simulink model "MPC"  (R2018a)
settings: Solver=VariableStepAuto  StartTime=0.0  StopTime=18  FixedStep=0.01  RelTol=1e-3
PreLoadFcn:
  | setUpPurePursuitCurveHighVel
model workspace (MAT data in the model file):
  firstWarning = 0
  originalScenarioChecksum = 'F73A6DA3C723D3CA73A6F931B7A52A9C'
values from neighbouring files (symbols this model uses):
  mu = m    [PSO_MPC.m]
  ref = i    [PSO_MPC.m]
  vx = j    [PSO_MPC.m]
  wy = l    [PSO_MPC.m]
undefined symbols (not defined in the file or in its folder): parms
libraries: autolibutils x4, autolibshared x3, vehdynlibviscommon x1, simulink x1
(part 1 of 3)
settings Model: PacingRate=0.700000  Creator=valakshe  LastModifiedBy=yassi
settings DataIOCC: ReturnWorkspaceOutputs=on
settings SFSimCC: SimUseLocalCustomCode=on
settings RTWCC: RTWUseLocalCustomCode=on

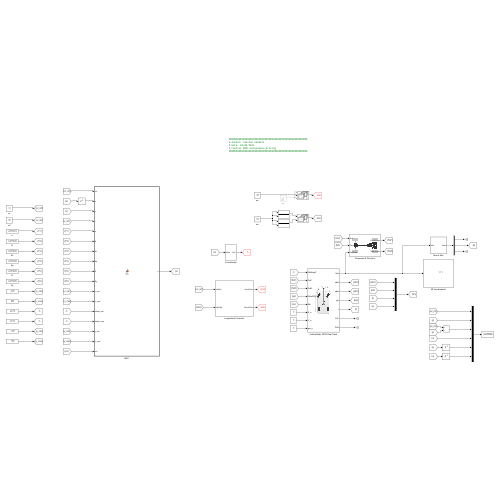
[thumbnail: Simulink's stored preview of the top-level diagram]
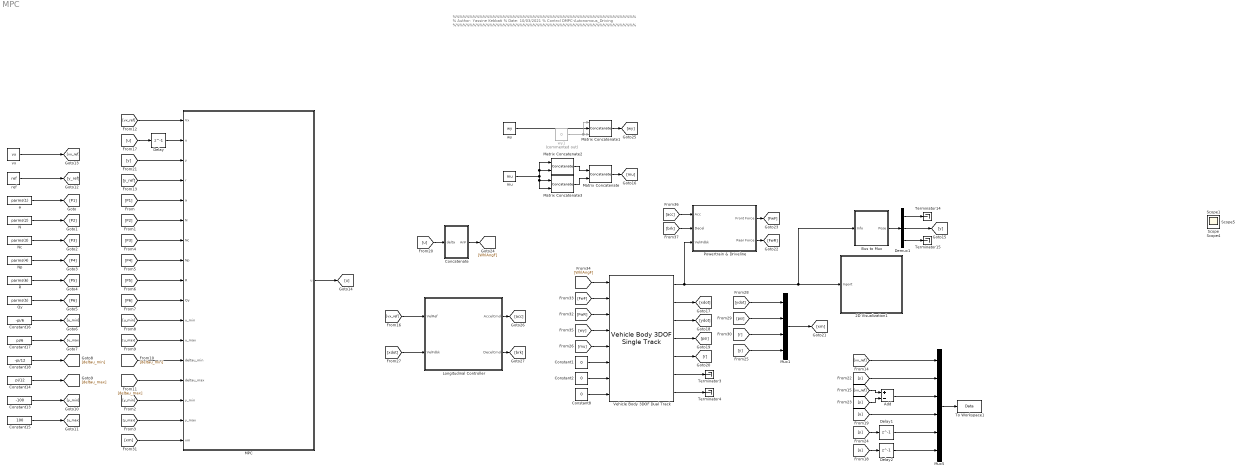
== system MPC ==
  note: %%%%%%%%%%%%%%%%%%%%%%%%%%%%%%%%%%%%%%%%%%%%%%%%%%%%%%%
      | % Author: Yassine Kebbati
      | % Date: 10/03/2021
      | % Control DMPC-Autonomous_Driving
      | %%%%%%%%%%%%%%%%%%%%%%%%%%%%%%%%%%%%%%%%%%%%%%%%%%%%%%%
  2D Visualization1 : Subsystem
      mask Display: image("visualization.JPG");
  Add : Sum  Inputs=+-
  Bus to Mux : Subsystem
  Concatenate : Subsystem
  Constant1 : Constant  Value=0
  Constant13 : Constant  Value=-100
  Constant14 : Constant  Value=pi/12
  Constant15 : Constant  Value=100
  Constant16 : Constant  Value=-pi/6
  Constant17 : Constant  Value=pi/6
  Constant18 : Constant  Value=-pi/12
  Constant2 : Constant  Value=0
  Constant8 : Constant  Value=0
  Delay : Delay  DelayLength=1
  Delay1 : Delay  DelayLength=1
  Delay2 : Delay  DelayLength=1
  Demux1 : Demux  Outputs=3
  Longitudinal Controller : Subsystem
  MPC : MATLAB Function  TreatAsAtomicUnit=on
  Matrix Concatenate : Concatenate  Mode=Multidimensional array  ConcatenateDimension=2
  Matrix Concatenate1 : Concatenate  NumInputs=3  Mode=Multidimensional array  ConcatenateDimension=2
  Matrix Concatenate2 : Concatenate  ConcatenateDimension=2
  Matrix Concatenate3 : Concatenate  ConcatenateDimension=2
  Mux1 : Mux
  Mux5 : Mux  Inputs=6
  N : Constant  Value=parms(2)
  Nc : Constant  Value=parms(3)
  Np : Constant  Value=parms(4)
  Powertrain & Driveline : Subsystem
      mask Display: image('vdbslibpt.png');
  Qy : Constant  Value=parms(5)
  R : Constant  Value=parms(6)
  Terminator{3..4,14..15} (4 alike) : Terminator
  To Workspace1 : ToWorkspace  VariableName=Data  SaveFormat=Timeseries  SampleTime=-1
  Vehicle Body 3DOF Dual Track : autolibshared/Vehicle Body 3DOF Single Track  trackMode=Dual  inputMode=External longitudinal forces  frontSteerMode=on  rearSteerMode=off  windMode=on  muMode=on  extFMode=off  extMMode=off  htchFMode=off  htchMMode=off  aMode=2  NF=2  NR=2  m=1575  a=1.2  b=1.6  h=0.35  dh=1  hh=0.2  X_o=0  xdot_o=0  CalphaMode=off  sigmaMode=on  hl=0  w=[1.4,1.4]  Cy_f=19e3  Cy_r=33e3  sigma_f=.1  sigma_r=.1  alpha_f_brk=[-.1 .1]  Cy_f_data=[-9e3 9e3]  alpha_r_brk=[-.1 .1]  Cy_r_data=[-9e3 9e3]  Y_o=0  ydot_o=0  Izz=2875  psi_o=0  r_o=0  Af=2  Cd=.3  Cl=.1  Cpm=.1  beta_w=[0:0.01:0.3]  Cs=[0:0.03:0.9]  Cym=[0:0.01:0.3]  Pabs=101325  Tair=273  g=9.81  mu=1  xdot_tol=0.01  Fznom=5000  Fxtire_sat=7e4  Fytire_sat=7e4
  a : Constant  Value=parms(1)
  mu : Constant  Value=mu
  ref : Constant  Value=ref
  vx : Constant  Value=vx
  wy : Constant  Value=wy
  wy1 : Constant  Commented=on  Value=0
  Scope{,1,4..5} (4 alike) : Scope
  wires:
  Vehicle Body 3DOF Dual Track/7 -> Terminator4/1
  Constant1/1 -> Vehicle Body 3DOF Dual Track/6
  Vehicle Body 3DOF Dual Track/6 -> Terminator3/1
  Constant2/1 -> Vehicle Body 3DOF Dual Track/7
  Constant8/1 -> Vehicle Body 3DOF Dual Track/8
  Vehicle Body 3DOF Dual Track/1 -> 2D Visualization1/1(Inport), Bus to Mux/1(Info), Powertrain & Driveline/3(VehFdbk)
  [acc] -> Powertrain & Driveline/1(Acc)
  [brk] -> Powertrain & Driveline/2(Decel)
  Vehicle Body 3DOF Dual Track/2 -> [xdot]
  Vehicle Body 3DOF Dual Track/4 -> [psi]
  Vehicle Body 3DOF Dual Track/5 -> [r]
  [P5] -> MPC/9(R)
  [P1] -> MPC/5(a)
  [P4] -> MPC/8(Np)
  [u_min] -> MPC/11(u_min)
  [deltau_min] -> MPC/13(deltau_min)
  [P3] -> MPC/7(Nc)
  [y_min] -> MPC/15(y_min)
  [y_max] -> MPC/16(y_max)
  Delay/1 -> MPC/2("u ")
  [deltau_max] -> MPC/14(deltau_max)
  [P2] -> MPC/6(N)
  [P6] -> MPC/10(Qy)
  [u_max] -> MPC/12(u_max)
  Demux1/3 -> Terminator15/1
  Demux1/1 -> Terminator14/1
  Vehicle Body 3DOF Dual Track/3 -> [ydot]
  Add/1 -> Mux5/3
  Mux5/1 -> To Workspace1/1
  Bus to Mux/1(Pose) -> Demux1/1
  Concatenate/1(AnF) -> [WhlAngF]
  wy/1 -> Matrix Concatenate1/2
  wy1/1 -> Matrix Concatenate1/1, Matrix Concatenate1/3
  Matrix Concatenate2/1 -> Matrix Concatenate/1
  mu/1 -> Matrix Concatenate2/1, Matrix Concatenate2/2, Matrix Concatenate3/1, Matrix Concatenate3/2
  Matrix Concatenate3/1 -> Matrix Concatenate/2
  Delay1/1 -> Mux5/5
  Delay2/1 -> Mux5/6
  Demux1/2 -> [y]
  a/1 -> [P1]
  N/1 -> [P2]
  Nc/1 -> [P3]
  Np/1 -> [P4]
  R/1 -> [P5]
  Qy/1 -> [P6]
  Constant16/1 -> [u_min]
  Constant17/1 -> [u_max]
  Constant18/1 -> [deltau_min]
  Constant14/1 -> [deltau_max]
  Constant13/1 -> [y_min]
  Constant15/1 -> [y_max]
  ref/1 -> [y_ref]
  vx/1 -> [vx_ref]
  [vx_ref] -> MPC/1(Vx)
  [y_ref] -> MPC/4(r)
  [vx_ref] -> Mux5/1
  [vx_ref] -> Add/1
  [vx_ref] -> Longitudinal Controller/1(VelRef)
  MPC/1(u) -> [u]
  [u] -> Delay/1
  [u] -> Delay2/1
  [u] -> Mux5/4
  [u] -> Concatenate/1(delta)
  [y] -> MPC/3(y)
  [y] -> Mux5/2
  [y] -> Add/2
  [y] -> Delay1/1
  [xdot] -> Longitudinal Controller/2(VelFdbk)
  [xm] -> MPC/17(xm)
  [psi] -> Mux1/2
  Mux1/1 -> [xm]
  [ydot] -> Mux1/1
  [r] -> Mux1/3
  [y] -> Mux1/4
  Powertrain & Driveline/2(Rear Force) -> [FwR]
  Powertrain & Driveline/1(Front Force) -> [FwF]
  [FwF] -> Vehicle Body 3DOF Dual Track/2
  [FwR] -> Vehicle Body 3DOF Dual Track/3
  [WhlAngF] -> Vehicle Body 3DOF Dual Track/1
  [mu] -> Vehicle Body 3DOF Dual Track/5
  Matrix Concatenate/1 -> [mu]
  [wy] -> Vehicle Body 3DOF Dual Track/4
  Matrix Concatenate1/1 -> [wy]
  Longitudinal Controller/1(AccelCmd) -> [acc]
  Longitudinal Controller/2(DecelCmd) -> [brk]

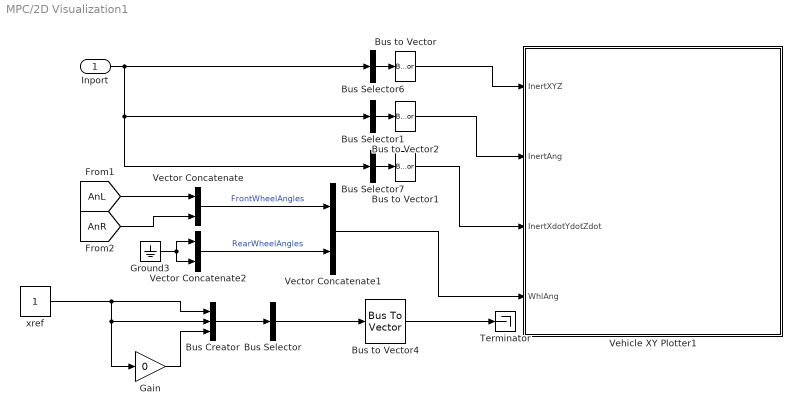
== system MPC/2D Visualization1 ==
  Inport : Inport
  Bus Creator : BusCreator  Inputs=3
  Bus Selector : BusSelector  OutputSignals=signal1,signal2,signal3  OutputAsBus=on
  Bus Selector1 : BusSelector  OutputSignals=InertFrm.Cg.Ang.phi,InertFrm.Cg.Ang.theta,InertFrm.Cg.Ang.psi  OutputAsBus=on
  Bus Selector6 : BusSelector  OutputSignals=InertFrm.Geom.Disp.X,InertFrm.Geom.Disp.Y,InertFrm.Geom.Disp.Z  OutputAsBus=on
  Bus Selector7 : BusSelector  OutputSignals=InertFrm.Geom.Vel.Xdot,InertFrm.Geom.Vel.Ydot,InertFrm.Geom.Vel.Zdot  OutputAsBus=on
  Bus to Vector{,1..2,4} (4 alike) : BusToVector
  Gain : Gain  Gain=0
  Ground3 : Ground
  Terminator : Terminator
  Vector Concatenate : Concatenate
  Vector Concatenate1 : Concatenate
  Vector Concatenate2 : Concatenate
  Vehicle XY Plotter1 : Subsystem  mask(Vehicle XY Plotter){extRef=off, extStats=off, extTireF=off, a=2, b=2, w=2, figBorder=10, bufferSize=1024, velNorm=5, tireFNorm=1000, pltDT=0.1}
      mask prompts: extRef "Plot path reference, extRef"; extStats "Display speed, RPM and Gear"; extTireF "Display tire forces"; a "Distance to front axle from CG, a [m]:"; b "Distance to rear axle from CG, b [m]:"; w "Track width, w [m]:"; figBorder "Distance to figure borders, figBorder [m]:"; bufferSize "Path buffer sampe size, bufferSize []:"; velNorm "Velocity vector scaling, velNorm [m*s/m]:"; tireFNorm "Tire force vector scaling, tireFNorm [m/N]:"; pltDT "Plot update rate, pltDT [s]:"
      mask help:
      | This block will display a MATLAB figure which indicates the vehicle path, current position and heading velocity.
      | An optional path reference is also provided.
      mask init:
      | block = gcb;
      | if autoblkschecksimstopped(block)
      |     ParamNames = {'extRef';'extStats';'extTireF';'extTireF'};
      |     PortNames = {'RefXYZ';'Stats';'TireFx';'TireFy'};
      |     for idx=1:length(PortNames)
      |         InportOption  = {'built-in/Ground', [PortNames{idx}, ' Ground'];...
      |             'built-in/Inport',PortNames{idx}};
      |         if ~strcmp(get_param(block,ParamNames{idx}),'on')
      |             NewBlkHdl = autoblksreplaceblock(block, InportOption, 1);
      |             set_param(NewBlkHdl, 'ShowName', 'off');
      |         else
      |             autoblksreplaceblock(block, InportOption, 2);
      |         end
      |     end
      |     InportNames = {'InertXYZ';'InertAng';'InertXdotYdotZdot';'WhlAng';'RefXYZ';'Stats';'TireFx';'TireFy'};
      |     FoundNames = get_param(find_system(block, 'LookUnderMasks', 'all', 'SearchDepth', 1, 'FollowLinks', 'on', 'BlockType', 'Inport'), 'Name');
      |     [~,PortI] = intersect(InportNames, FoundNames);
      |     PortI = sort(PortI);
      |     for idx = 1:length(PortI)
      |         set_param([block, '/', InportNames{PortI(idx)}], 'Port', num2str(idx));
      |     end
      | end
      mask TypeOptions a: Vehicle XY Plotter/a
      mask TypeOptions b: Vehicle XY Plotter/b
      mask TypeOptions w: Vehicle XY Plotter/w
      mask TypeOptions figBorder: Vehicle XY Plotter/figBorder
      mask TypeOptions bufferSize: Vehicle XY Plotter/bufferSize
      mask TypeOptions velNorm: Vehicle XY Plotter/velNorm
      mask TypeOptions tireFNorm: Vehicle XY Plotter/tireFNorm
      mask DialogControl Container3 Prompt: Plot and Display Options
  xref : Constant
  wires:
  Vector Concatenate1/1 -> Vehicle XY Plotter1/4(WhlAng)
  Ground3/1 -> Vector Concatenate2/1, Vector Concatenate2/2
  Bus Selector6/1 -> Bus to Vector/1
  Vector Concatenate/1 -> Vector Concatenate1/1  "FrontWheelAngles"
  [AnL] -> Vector Concatenate/1
  Vector Concatenate2/1 -> Vector Concatenate1/2  "RearWheelAngles"
  Bus Selector7/1 -> Bus to Vector1/1
  Bus to Vector1/1 -> Vehicle XY Plotter1/3(InertXdotYdotZdot)
  Bus to Vector/1 -> Vehicle XY Plotter1/1(InertXYZ)
  Bus to Vector2/1 -> Vehicle XY Plotter1/2(InertAng)
  Bus Selector1/1 -> Bus to Vector2/1
  [AnR] -> Vector Concatenate/2
  Inport/1 -> Bus Selector7/1, Bus Selector1/1, Bus Selector6/1
  Bus to Vector4/1 -> Terminator/1
  Bus Selector/1 -> Bus to Vector4/1
  xref/1 -> Gain/1, Bus Creator/2, Bus Creator/1
  Gain/1 -> Bus Creator/3
  Bus Creator/1 -> Bus Selector/1

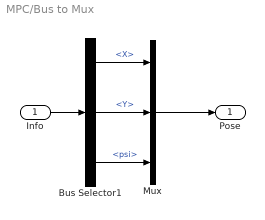
== system MPC/Bus to Mux ==
  Info : Inport
  Bus Selector1 : BusSelector  OutputSignals=InertFrm.Cg.Disp.X,InertFrm.Cg.Disp.Y,InertFrm.Cg.Ang.psi
  Mux : Mux  Inputs=3
  Pose : Outport
  wires:
  Bus Selector1/3 -> Mux/3  "<psi>"
  Bus Selector1/1 -> Mux/1  "<X>"
  Mux/1 -> Pose/1
  Bus Selector1/2 -> Mux/2  "<Y>"
  Info/1 -> Bus Selector1/1

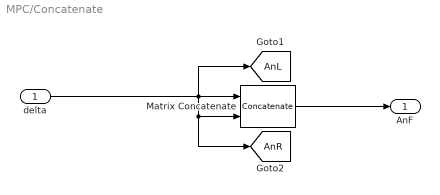
== system MPC/Concatenate ==
  delta : Inport
  Matrix Concatenate : Concatenate
  AnF : Outport  VectorParamsAs1DForOutWhenUnconnected=off
  tag scope: AnL=global, AnR=global
  wires:
  Matrix Concatenate/1 -> AnF/1
  delta/1 -> [AnL], [AnR], Matrix Concatenate/2, Matrix Concatenate/1

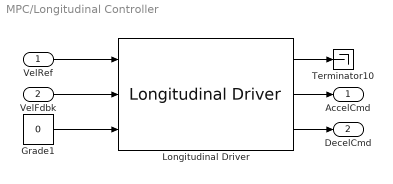
== system MPC/Longitudinal Controller ==
  VelRef : Inport
  VelFdbk : Inport  Port=2
  Grade1 : Constant  Value=0
  Longitudinal Driver : autolibshared/Longitudinal Driver  Kp=100  Ki=1  Kff=.1  Kg=0  vnom=9  Kaw=1  tauerr=.01  aMode=2
  Terminator10 : Terminator
  AccelCmd : Outport
  DecelCmd : Outport  Port=2
  wires:
  Grade1/1 -> Longitudinal Driver/3
  Longitudinal Driver/3 -> DecelCmd/1
  VelRef/1 -> Longitudinal Driver/1
  VelFdbk/1 -> Longitudinal Driver/2
  Longitudinal Driver/2 -> AccelCmd/1
  Longitudinal Driver/1 -> Terminator10/1

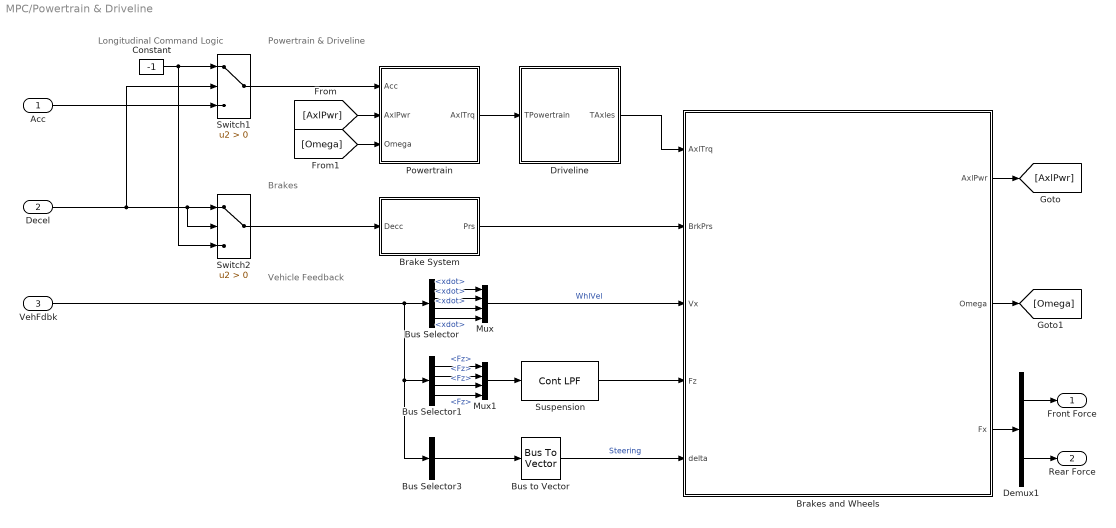
== system MPC/Powertrain & Driveline ==
  note: Vehicle Feedback
  note: Powertrain & Driveline
  note: Brakes
  note: Longitudinal Command Logic
  Acc : Inport
  Decel : Inport  Port=2
  VehFdbk : Inport  Port=3
  Brake System : Subsystem
  Brakes and Wheels : Subsystem  TreatAsAtomicUnit=on
      mask Display: image('vdbslibwhls.png');
  Bus Selector : BusSelector  OutputSignals=BdyFrm.FrntAxl.Lft.Vel.xdot,BdyFrm.FrntAxl.Rght.Vel.xdot,BdyFrm.RearAxl.Lft.Vel.xdot,BdyFrm.RearAxl.Rght.Vel.xdot
  Bus Selector1 : BusSelector  OutputSignals=BdyFrm.Forces.FrntAxl.Lft.Fz,BdyFrm.Forces.FrntAxl.Rght.Fz,BdyFrm.Forces.RearAxl.Lft.Fz,BdyFrm.Forces.RearAxl.Rght.Fz
  Bus Selector3 : BusSelector  OutputSignals=BdyFrm.FrntAxl.Steer.WhlAngFL,BdyFrm.FrntAxl.Steer.WhlAngFR,BdyFrm.RearAxl.Steer.WhlAngRL,BdyFrm.RearAxl.Steer.WhlAngRR  OutputAsBus=on
  Bus to Vector : BusToVector
  Constant : Constant  Value=-1
  Demux1 : Demux  Outputs=[2 2]
  Driveline : Subsystem  Variant=on  VariantControl=Variant1  OverrideUsingVariant=0
  Mux : Mux
  Mux1 : Mux
  Powertrain : Subsystem
  Suspension : autolibutils/Cont LPF  wc=10*pi*2  AbsoluteTolerance=auto  aMode=2
  Switch1 : Switch  Criteria=u2 > Threshold
  Switch2 : Switch  Criteria=u2 > Threshold
  Front Force : Outport  VectorParamsAs1DForOutWhenUnconnected=off
  Rear Force : Outport  Port=2  VectorParamsAs1DForOutWhenUnconnected=off
  wires:
  Brake System/1(Prs) -> Brakes and Wheels/2(BrkPrs)
  Switch2/1 -> Brake System/1(Decc)
  [Omega] -> Powertrain/3(Omega)
  [AxlPwr] -> Powertrain/2(AxlPwr)
  Brakes and Wheels/2(Omega) -> [Omega]
  Powertrain/1(AxlTrq) -> Driveline/1(TPowertrain)
  Switch1/1 -> Powertrain/1(Acc)
  Bus Selector1/4 -> Mux1/4  "<Fz>"
  Bus Selector1/3 -> Mux1/3  "<Fz>"
  Bus Selector1/2 -> Mux1/2  "<Fz>"
  Bus Selector1/1 -> Mux1/1  "<Fz>"
  Bus Selector/4 -> Mux/4  "<xdot>"
  Bus Selector/3 -> Mux/3  "<xdot>"
  Bus Selector/2 -> Mux/2  "<xdot>"
  Bus Selector/1 -> Mux/1  "<xdot>"
  Suspension/1 -> Brakes and Wheels/4(Fz)
  Mux1/1 -> Suspension/1
  Bus to Vector/1 -> Brakes and Wheels/5(delta)  "Steering"
  Bus Selector3/1 -> Bus to Vector/1
  Brakes and Wheels/3(Fx) -> Demux1/1
  Brakes and Wheels/1(AxlPwr) -> [AxlPwr]
  Driveline/1(TAxles) -> Brakes and Wheels/1(AxlTrq)
  Demux1/2 -> Rear Force/1
  Demux1/1 -> Front Force/1
  VehFdbk/1 -> Bus Selector/1, Bus Selector1/1, Bus Selector3/1
  Mux/1 -> Brakes and Wheels/3(Vx)  "WhlVel"
  Constant/1 -> Switch1/1, Switch2/3
  Acc/1 -> Switch1/3
  Decel/1 -> Switch2/1, Switch2/2, Switch1/2

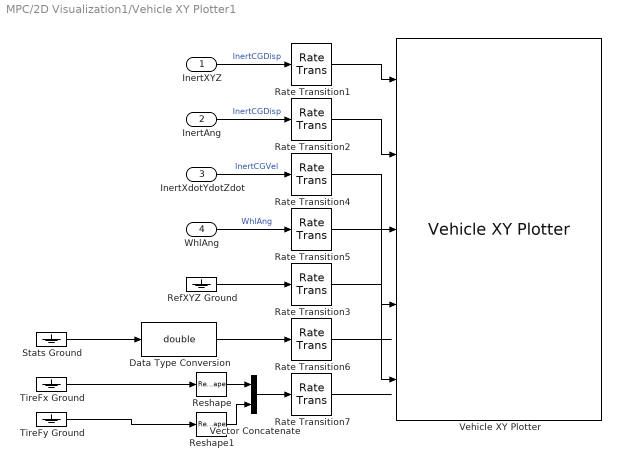
== system MPC/2D Visualization1/Vehicle XY Plotter1 ==
  InertXYZ : Inport
  InertAng : Inport  Port=2
  InertXdotYdotZdot : Inport  Port=3
  WhlAng : Inport  Port=4
  Data Type Conversion : DataTypeConversion  OutDataTypeStr=double
  Rate Transition{1..7} (7 alike) : RateTransition  Deterministic=off  OutPortSampleTime=pltDT
  RefXYZ Ground : Ground
  Reshape : Reshape  OutputDimensionality=Row vector (2-D)
  Reshape1 : Reshape  OutputDimensionality=Row vector (2-D)
  Stats Ground : Ground
  TireFx Ground : Ground
  TireFy Ground : Ground
  Vector Concatenate : Concatenate  Mode=Multidimensional array
  Vehicle XY Plotter : vehdynlibviscommon/Vehicle XY Plotter  w=w  a=a  b=b  figBorder=figBorder  bufferSize=bufferSize
  wires:
  Vector Concatenate/1 -> Rate Transition7/1
  Reshape1/1 -> Vector Concatenate/2
  Reshape/1 -> Vector Concatenate/1
  Rate Transition7/1 -> ?
  Data Type Conversion/1 -> Rate Transition6/1
  Rate Transition6/1 -> ?
  Rate Transition5/1 -> Vehicle XY Plotter/4
  Rate Transition4/1 -> Vehicle XY Plotter/3
  Rate Transition2/1 -> Vehicle XY Plotter/2
  Rate Transition1/1 -> Vehicle XY Plotter/1
  Rate Transition3/1 -> Vehicle XY Plotter/5
  WhlAng/1 -> Rate Transition5/1  "WhlAng"
  InertXYZ/1 -> Rate Transition1/1  "InertCGDisp"
  InertXdotYdotZdot/1 -> Rate Transition4/1  "InertCGVel"
  InertAng/1 -> Rate Transition2/1  "InertCGDisp"
  TireFx Ground/1 -> Reshape/1
  TireFy Ground/1 -> Reshape1/1
  Stats Ground/1 -> Data Type Conversion/1
  RefXYZ Ground/1 -> Rate Transition3/1

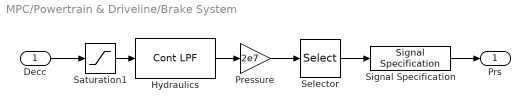
== system MPC/Powertrain & Driveline/Brake System ==
  Decc : Inport
  Hydraulics : autolibutils/Cont LPF  wc=30*pi*2  AbsoluteTolerance=auto  aMode=2
  Pressure : Gain  Gain=2e7
  Saturation1 : Saturate  UpperLimit=inf  LowerLimit=0  ZeroCross=off
  Selector : Selector  InputPortWidth=1  IndexOptions=Index vector (dialog)  Indices=[1 1 1 1]  OutputSizes=1
  Signal Specification : SignalSpecification  Unit=Pa
  Prs : Outport  VectorParamsAs1DForOutWhenUnconnected=off
  wires:
  Signal Specification/1 -> Prs/1
  Decc/1 -> Saturation1/1
  Selector/1 -> Signal Specification/1
  Saturation1/1 -> Hydraulics/1
  Hydraulics/1 -> Pressure/1
  Pressure/1 -> Selector/1
